simulink model "HW6_F"  (R2018a)
settings: Solver=VariableStepAuto  StartTime=0.0  StopTime=20  RelTol=1e-3
StartFcn:
  | vtol_param
  | HW6_F_new
undefined symbols (not defined in the file or in its folder): K, p, P, PlotVtol, z
settings Model: Creator=sadam  LastModifiedBy=sadam

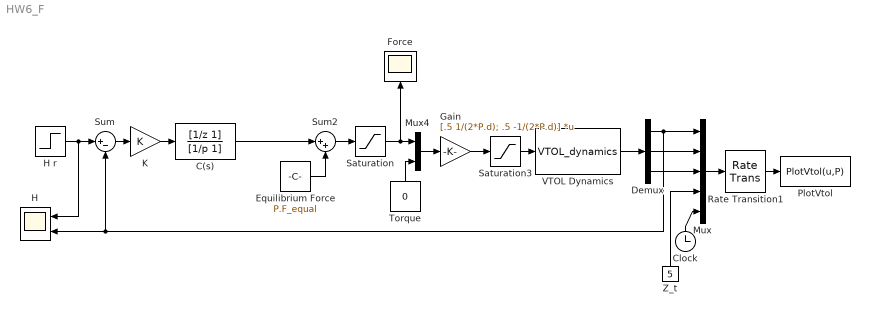
== system HW6_F ==
  C(s) : TransferFcn  Numerator=[1/z 1]  Denominator=[1/p 1]
  Clock : Clock
  Demux : Demux  Outputs=3
  Equilibrium Force : Constant  Value=P.F_equal
  "Force " : Scope
  Gain : Gain  Gain=[.5 1/(2*P.d); .5 -1/(2*P.d)]  Multiplication=Matrix(K*u)
  "H " : Scope  NumInputPorts=2
  H r : Step  SampleTime=0
  K : Gain  Gain=K
  Mux : Mux  Inputs=5
  Mux4 : Mux  Inputs=2
  "PlotVtol " : MATLABFcn  MATLABFcn=PlotVtol(u,P)  OutputDimensions=0
  Rate Transition1 : RateTransition  OutPortSampleTime=P.t_plot
  Saturation : Saturate  UpperLimit=P.Force_max  LowerLimit=-P.Force_max
  Saturation3 : Saturate  UpperLimit=P.Force_max  LowerLimit=-P.Force_max
  Sum : Sum  Inputs=|+-
  Sum2 : Sum  Inputs=|++
  Torque : Constant  Value=0
  VTOL Dynamics : S-Function  FunctionName=VTOL_dynamics  Parameters=P  SFunctionDeploymentMode=off  EnableBusSupport=off
  Z_t : Constant  Value=5
  wires:
  Demux/2 -> Mux/2
  Demux/3 -> Mux/3
  Demux/1 -> "H "/2, Sum/2, Mux/1
  Saturation3/1 -> VTOL Dynamics/1
  Rate Transition1/1 -> "PlotVtol "/1
  Mux/1 -> Rate Transition1/1
  Clock/1 -> Mux/5
  Z_t/1 -> Mux/4
  VTOL Dynamics/1 -> Demux/1
  Mux4/1 -> Gain/1
  Gain/1 -> Saturation3/1
  K/1 -> C(s)/1
  Torque/1 -> Mux4/2
  H r/1 -> "H "/1, Sum/1
  Sum/1 -> K/1
  Equilibrium Force/1 -> Sum2/2
  Sum2/1 -> Saturation/1
  Saturation/1 -> "Force "/1, Mux4/1
  C(s)/1 -> Sum2/1
